simulink model "MIL_Model"  (R2024b)
settings: Solver=FixedStepDiscrete  StartTime=0.0  StopTime=10  FixedStep=50e-6  RelTol=1e-3
InitFcn:
  | PID_Data;
values from neighbouring files (symbols this model uses):
  Test_Speed_RPM = 1000    [PID_Data.m]    (also in PMSM_PID_Data.m)
settings Model: Creator=BitCore  LastModifiedBy=BitCore

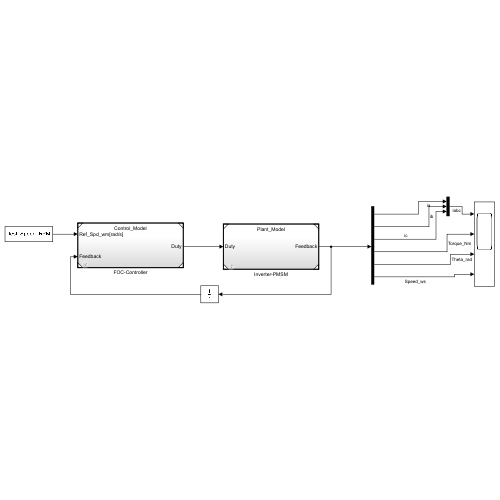
[thumbnail: Simulink's stored preview of the top-level diagram]
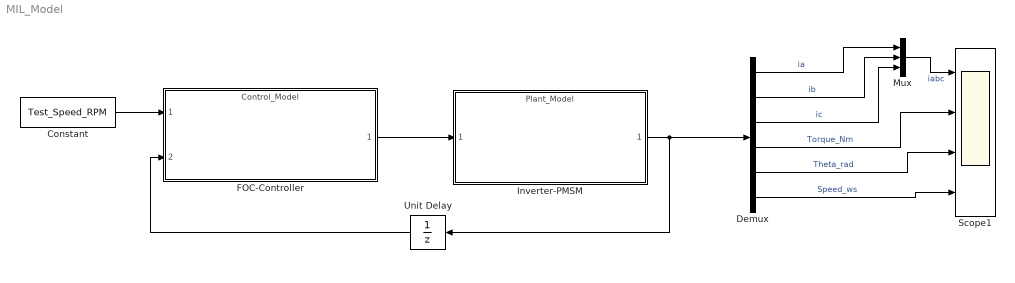
== system MIL_Model ==
  Constant : Constant  Value=Test_Speed_RPM  OutDataTypeStr=single
  Demux : Demux  Outputs=6
  FOC-Controller : ModelReference  ModelNameDialog=Control_Model.slx  SimulationMode=Normal  ModelReferenceVersion=1.96
  Inverter-PMSM : ModelReference  ModelNameDialog=Plant_Model.slx  SimulationMode=Normal  ModelReferenceVersion=1.56
  Mux : Mux  Inputs=3
  Scope1 : Scope  NumInputPorts=4
  Unit Delay : UnitDelay  SampleTime=-1  HasFrameUpgradeWarning=on
  wires:
  Constant/1 -> FOC-Controller/1
  Demux/1 -> Mux/1  "ia"
  Demux/2 -> Mux/2  "ib"
  Demux/3 -> Mux/3  "ic"
  Demux/4 -> Scope1/2  "Torque_Nm"
  Demux/5 -> Scope1/3  "Theta_rad"
  Demux/6 -> Scope1/4  "Speed_ws"
  Unit Delay/1 -> FOC-Controller/2
  Mux/1 -> Scope1/1  "iabc"
  Inverter-PMSM/1 -> Unit Delay/1, Demux/1
  FOC-Controller/1 -> Inverter-PMSM/1
